simulink model "subRangeModule"  (R2024b)
settings: Solver=VariableStepAuto  StartTime=0.0  StopTime=10.0  RelTol=1e-3
values from neighbouring files (symbols this model uses):
  B1 = 4    [TestWrapper.m]
  C_f1 = C_s/G1    (= 2.5e-10)    [TestWrapper.m]
  C_s = 2000000e-15    (= 2e-09)    [TestWrapper.m]
  C_samp = 1000000e-15    (= 1e-09)    [TestWrapper.m]
  FSR = 2.4    [TestWrapper.m]
  G1 = 2^(B1-1)    (= 8)    [TestWrapper.m]
  k = 1.38e-23    [TestWrapper.m]
  LGBW = 60*fs    (= 18000000000)    [TestWrapper.m]
  R_sw = .01    (= 0.01)    [TestWrapper.m]
  T = 300    [TestWrapper.m]
  ts = 1/fs    (= 3.33333333333e-09)    [TestWrapper.m]
  Vt_offset_en = true    [TestWrapper.m]
  Vt_var = 0.01    [TestWrapper.m]
libraries: dspsrcs4 x2
settings Model: Creator=bbassett6  LastModifiedBy=bbassett6

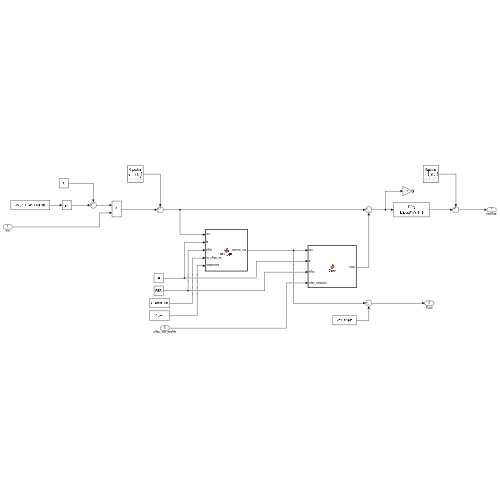
[thumbnail: Simulink's stored preview of the top-level diagram]
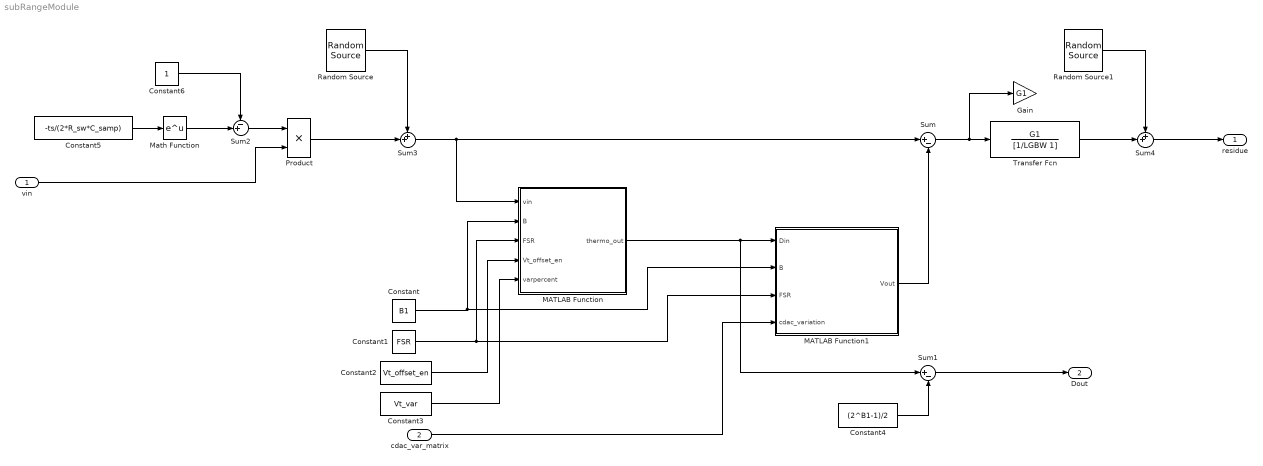
== system subRangeModule ==
  vin : Inport
  cdac_var_matrix : Inport  Port=2
  Constant : Constant  Value=B1
  Constant1 : Constant  Value=FSR
  Constant2 : Constant  Value=Vt_offset_en
  Constant3 : Constant  Value=Vt_var
  Constant4 : Constant  Value=(2^B1-1)/2
  Constant5 : Constant  Value=-ts/(2*R_sw*C_samp)
  Constant6 : Constant
  Gain : Gain  Gain=G1
  MATLAB Function : MATLAB Function  TreatAsAtomicUnit=on
  MATLAB Function1 : MATLAB Function  TreatAsAtomicUnit=on
  Math Function : Math
  Product : Product
  Random Source : dspsrcs4/Random Source  SrcType=Gaussian  MinVal=0  MaxVal=1  MeanVal=0  VarVal=k*T/C_samp  RepMode=Not repeatable  rawSeed=1  IsInherit=off  SampTime=1  SampFrame=1  OutComplex=Real  DataType=double  SimulateUsing=Interpreted execution
  Random Source1 : dspsrcs4/Random Source  SrcType=Gaussian  MinVal=0  MaxVal=1  MeanVal=0  VarVal=2*k*T*(C_s+C_f1)/C_f1^2  RepMode=Not repeatable  rawSeed=1  IsInherit=off  SampTime=1  SampFrame=1  OutComplex=Real  DataType=double  SimulateUsing=Interpreted execution
  Sum : Sum  Inputs=|+-
  Sum1 : Sum  Inputs=|+-
  Sum2 : Sum  Inputs=-+|
  Sum3 : Sum  Inputs=++|
  Sum4 : Sum  Inputs=++|
  Transfer Fcn : TransferFcn  Numerator=G1  Denominator=[1/LGBW 1]
  residue : Outport
  Dout : Outport  Port=2
  wires:
  Sum2/1 -> Product/1
  Transfer Fcn/1 -> Sum4/2
  Constant2/1 -> MATLAB Function/4(Vt_offset_en)
  Sum3/1 -> MATLAB Function/1(vin), Sum/1
  Random Source/1 -> Sum3/1
  MATLAB Function/1(thermo_out) -> Sum1/1, MATLAB Function1/1(Din)
  Sum1/1 -> Dout/1
  Constant1/1 -> MATLAB Function1/3(FSR), MATLAB Function/3(FSR)
  MATLAB Function1/1(Vout) -> Sum/2
  Constant/1 -> MATLAB Function1/2(B), MATLAB Function/2(B)
  Random Source1/1 -> Sum4/1
  Constant3/1 -> MATLAB Function/5(varpercent)
  cdac_var_matrix/1 -> MATLAB Function1/4(cdac_variation)
  Sum/1 -> Transfer Fcn/1, Gain/1
  vin/1 -> Product/2
  Constant4/1 -> Sum1/2
  Constant6/1 -> Sum2/1
  Math Function/1 -> Sum2/2
  Constant5/1 -> Math Function/1
  Product/1 -> Sum3/2
  Sum4/1 -> residue/1

== matlab function subRangeModule/MATLAB Function1 ==
  data: Din input; Vout output size=1; B input; FSR input; cdac_variation input
function Vout = Cdac(Din, B, FSR, cdac_variation)

% LSB = FSR/2^B;

y = [1 1 2 4 8 16 32 64 128 256 512 1024 2048 4096];

Cdac_array = y(1:B+1).*cdac_variation(1:B+1);
Cdac_array = flip(Cdac_array);

Dout = dec2bin(Din*2,B+1);
Dout_num = ones(length(Dout),1);

for n=1:length(Dout)
    if abs(str2double(Dout(n)))==1
        Dout_num(n) = abs(str2double(Dout(n)));
    else
        Dout_num(n) = -1;
    end
end
Dout_num(B+1) = 0;
Dout_num;
VOUT = Cdac_array*Dout_num/(sum(Cdac_array));
Vout = sum(VOUT*FSR/2);
% VOUT = cast(Vout, "double");
% Cdac.outputs(1).DataType = 'double';

end

== matlab function subRangeModule/MATLAB Function ==
  data: vin input; thermo_out output; B input; FSR input; Vt_offset_en input; varpercent input
function thermo_out = flash_qtz(vin, B, FSR, Vt_offset_en, varpercent)

LSB = FSR/2^B;

variation = rand(1,2^B-1);
variation = variation-0.5;
variation = variation.*varpercent;
vt_variation = variation+1;

Vtrans = -FSR/2+LSB:LSB:FSR/2-LSB;

if Vt_offset_en
    Vtrans = Vtrans + 0.01*Vtrans.^2 + 0.01*Vtrans.^3;
end

Vtrans = Vtrans.*vt_variation;

thermo_out = sum(vin>Vtrans);

end
